simulink model "Radial_LV_Grid_Third"  (R2022a)
settings: Solver=ode23t  StartTime=0.0  StopTime=2  MaxStep=0.1  RelTol=1e-3
libraries: spsThreePhaseVIMeasurementLib x5, spsLoadFlowBusLib x4, spsPower3phPhasorLib x4, spsThreePhaseDynamicLoadLib x3, spsThreePhasePISectionLineLib x2, spsThreePhaseSourceLib x1, spsThreePhaseTransformerTwoWindingsLib x1, spspowerguiLib x1
settings Model: Creator=matm  LastModifiedBy=nikos
settings SolverCC: ShapePreserveControl=EnableAll  AlgebraicLoopSolver=TrustRegion  SolverResetMethod=Robust
settings DataIOCC: ReturnWorkspaceOutputs=off
settings DebuggingCC: SFMachineParentedDataDiag=warning  ArithmeticOperatorsInVariantConditions=warning
settings SFSimCC: SimUseLocalCustomCode=off  CustomCodeUndefinedFunction=UseInterfaceOnly
settings RTWCC: RTWUseLocalCustomCode=off
settings CodeAppCC: StateflowObjectComments=on
settings SimscapeCC: SimscapeNormalizeSystem=off

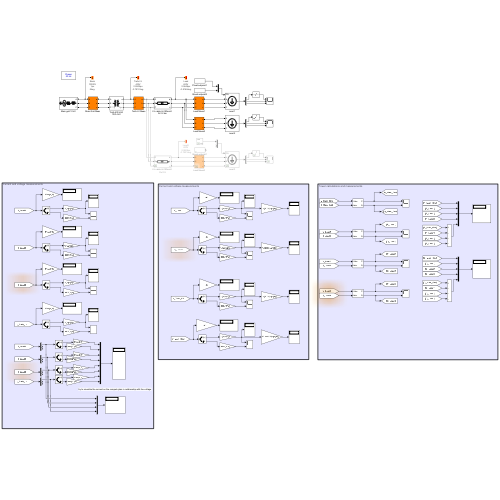
[thumbnail: Simulink's stored preview of the top-level diagram]
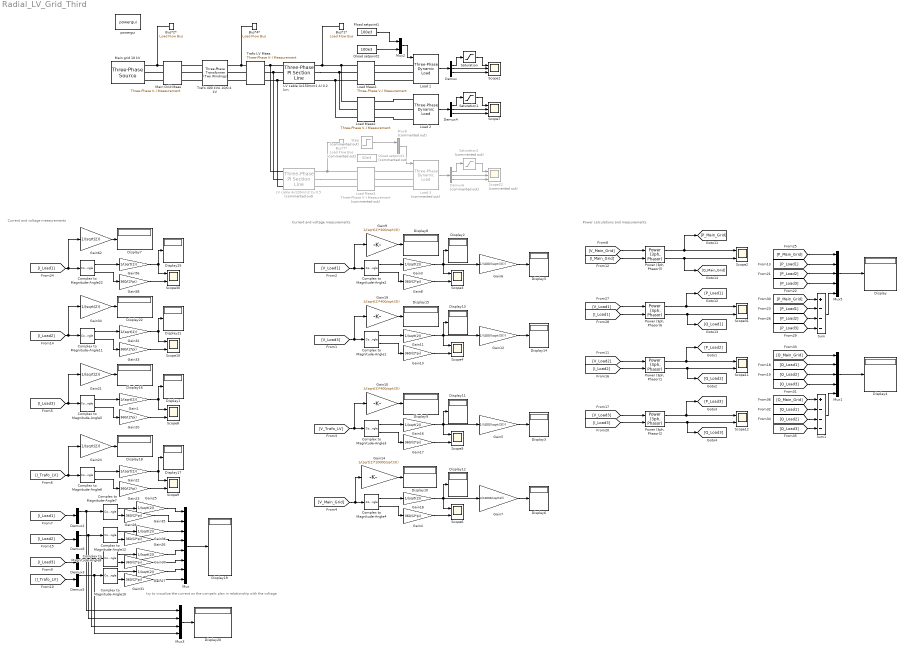
== system Radial_LV_Grid_Third ==
  note: try to visualize the current on the compelx plan in relationship with the voltage
  note: Current and voltage measurements
  note: Power calculations and measurements
  note: Current and voltage measurements
  Bus*1* : spsLoadFlowBusLib/Load Flow Bus  LConnTagsString=a  Phases=single  Connectors=on one side  ID=Load  Vbase=400  Vref=1  Vangle=0  VLF=0.9446  VLFb=1  VLFc=1  angleLF=-0.8162  angleLFb=0  angleLFc=0
      settings: SourceProductBaseCode=PS
  Bus*2* : spsLoadFlowBusLib/Load Flow Bus  LConnTagsString=a  Phases=single  Connectors=on one side  ID=Slack  Vbase=10000  Vref=1  Vangle=0  VLF=1  VLFb=1  VLFc=1  angleLF=0  angleLFb=0  angleLFc=0
      settings: SourceProductBaseCode=PS
  Bus*4* : spsLoadFlowBusLib/Load Flow Bus  LConnTagsString=a  Phases=single  Connectors=on one side  ID=Trafo LV  Vbase=400  Vref=1  Vangle=0  VLF=0.9905  VLFb=1  VLFc=1  angleLF=-0.7817  angleLFb=0  angleLFc=0
      settings: SourceProductBaseCode=PS
  Bus*7* : spsLoadFlowBusLib/Load Flow Bus  Commented=on  LConnTagsString=a  Phases=single  Connectors=on one side  ID=Load3  Vbase=400  Vref=1  Vangle=0  VLF=0.9905  VLFb=1  VLFc=1  angleLF=-0.7821  angleLFb=0  angleLFc=0
      settings: SourceProductBaseCode=PS
  Complex to Magnitude-Angle{1..8,10..12,22} (12 alike) : ComplexToMagnitudeAngle
  Demux{,2..5,8} (6 alike) : Demux  Outputs=3
  Demux6 : Demux  Commented=on  Outputs=3
  Display{,1..22,25} (24 alike) : Display
  Gain{1,3,11,16,18,21..22,24..27,32,34..35,56,62} (16 alike) : Gain  Gain=1/(sqrt(2))
  Gain10 : Gain  Gain=1/(sqrt(2)*400/sqrt(3))
  Gain12 : Gain  Gain=1/(400/(sqrt(3)))
  Gain{4,8,13,17,20,23,28,30..31,33,36,58} (12 alike) : Gain  Gain=360/(2*pi)
  Gain14 : Gain  Gain=1/(sqrt(2)*10000/sqrt(3))
  Gain19 : Gain  Gain=1/(sqrt(2)*400/sqrt(3))
  Gain5 : Gain  Gain=1/(400/(sqrt(3)))
  Gain6 : Gain  Gain=1/(400/(sqrt(3)))
  Gain7 : Gain  Gain=1/(10000/(sqrt(3)))
  Gain9 : Gain  Gain=1/(sqrt(2)*400/sqrt(3))
  LV cable 4x120mm2 Cu 0.5 : spsThreePhasePISectionLineLib/Three-Phase PI Section Line  Commented=on  LConnTagsString=a|b|c  RConnTagsString=A|B|C  Length=0.5  Frequency=50  Resistances=[ 0.1556 0.6224]  Inductances=[ 72e-3/(2*pi*50) 288e-3/(2*pi*50)]  Capacitances=[910e-09 455e-09]
  LV cable 4x150mm2 Al 0.2 km : spsThreePhasePISectionLineLib/Three-Phase PI Section Line  LConnTagsString=a|b|c  RConnTagsString=A|B|C  Length=0.2  Frequency=50  Resistances=[ 0.207 0.828]  Inductances=[ 72e-3/(2*pi*50) 288e-3/(2*pi*50)]  Capacitances=[910e-09 455e-09]
  Load 1 : spsThreePhaseDynamicLoadLib/Three-Phase Dynamic Load  NominalVoltage=[ 0.4e3 50 ]  ActiveReactivePowers=[100000 100e3]  PositiveSequence=[0.944639 -0.816214]  ExternalControl=on  NpNq=[0 0]  TimeConstants="[0  0  0  0]"  MinimumVoltage=0.7  Tfilter=1e-4  LoadFlowParameters=[4 100000 0 0 100000]
      settings: SourceProductBaseCode=PS
  Load 2 : spsThreePhaseDynamicLoadLib/Three-Phase Dynamic Load  NominalVoltage=[ 0.4e3 50 ]  ActiveReactivePowers=[50000 50000]  PositiveSequence=[0.944639 -0.816214]  ExternalControl=off  NpNq=[1 2]  TimeConstants="[0  0  0  0]"  MinimumVoltage=0.7  Tfilter=1e-4  LoadFlowParameters=[4 100000 0 0 100000]
      settings: SourceProductBaseCode=PS
  Load 3 : spsThreePhaseDynamicLoadLib/Three-Phase Dynamic Load  Commented=on  NominalVoltage=[ 0.4e3 50 ]  ActiveReactivePowers=[0 0]  PositiveSequence=[0.990467 -0.782078]  ExternalControl=on  NpNq=[0 0]  TimeConstants="[0  0  0  0]"  MinimumVoltage=0.7  Tfilter=1e-4  LoadFlowParameters=[4 100000 0 0 100000]
      settings: SourceProductBaseCode=PS
  Load Meas1 : spsThreePhaseVIMeasurementLib/Three-Phase V-I Measurement  VoltageMeasurement=phase-to-ground  SetLabelV=on  LabelV=V_Load1  Vpu=off  VpuLL=off  CurrentMeasurement=yes  SetLabelI=on  LabelI=I_Load1  Ipu=off  Pbase=100e6  Vbase=500e3  OutputType=Complex  PhasorSimulation=on  PSBequivalent=0
  Load Meas2 : spsThreePhaseVIMeasurementLib/Three-Phase V-I Measurement  VoltageMeasurement=phase-to-ground  SetLabelV=on  LabelV=V_Load2  Vpu=off  VpuLL=off  CurrentMeasurement=yes  SetLabelI=on  LabelI=I_Load2  Ipu=off  Pbase=100e6  Vbase=500e3  OutputType=Complex  PhasorSimulation=on  PSBequivalent=0
  Load Meas3 : spsThreePhaseVIMeasurementLib/Three-Phase V-I Measurement  Commented=on  VoltageMeasurement=phase-to-ground  SetLabelV=on  LabelV=V_Load3  Vpu=off  VpuLL=off  CurrentMeasurement=yes  SetLabelI=on  LabelI=I_Load3  Ipu=off  Pbase=100e6  Vbase=500e3  OutputType=Complex  PhasorSimulation=on  PSBequivalent=0
  Main Grid Meas : spsThreePhaseVIMeasurementLib/Three-Phase V-I Measurement  VoltageMeasurement=phase-to-ground  SetLabelV=on  LabelV=V_Main_Grid  Vpu=off  VpuLL=off  CurrentMeasurement=yes  SetLabelI=on  LabelI=I_Main_Grid  Ipu=off  Pbase=100e6  Vbase=500e3  OutputType=Complex  PhasorSimulation=on  PSBequivalent=0
  Main grid 10 kV : spsThreePhaseSourceLib/Three-Phase Source  InternalConnection=Yg  VoltagePhases=off  Voltage=(10000)*1.0073  PhaseAngle=0.871  Voltage_phases=[25e3 25e3 25e3]/sqrt(3)  PhaseAngles_phases=[0 -120 +120]  Frequency=50  NonIdealSource=on  SpecifyImpedance=on  Resistance=0.8929  Inductance=16.58e-3  ShortCircuitLevel=10e6  BaseVoltage=10e3  XRratio=10  BusType=swing  Pref=10e3  Qref=0  Prefabc=[10e3, 10e3, 10e3]  Qrefabc=[0, 0, 0]  Qmin=-inf  Qmax=inf
  Mux : Mux  Inputs=8
  Mux1 : Mux  Inputs=5
  Mux2 : Mux  Inputs=2
  Mux3 : Mux
  Mux5 : Mux  Inputs=5
  Mux8 : Mux  Commented=on  Inputs=2
  Pload setpoint1 : Constant  Value=100e3
  Power (3ph, Phasor){1..2,5..6} (4 alike) : spsPower3phPhasorLib/Power (3ph, Phasor)
      settings: SourceProductBaseCode=PS
  Qload setpoint1 : Constant  Commented=on  Value=50e3
  Qload setpoint2 : Constant  Value=100e3
  Saturation : Saturate  UpperLimit=1.15  LowerLimit=0.85
  Saturation1 : Saturate  UpperLimit=1.15  LowerLimit=0.85
  Saturation2 : Saturate  Commented=on  UpperLimit=1.15  LowerLimit=0.85
  Scope1 : Scope  NumInputPorts=3
  Scope{2..6,8..12,30..31} (12 alike) : Scope  NumInputPorts=2
  Scope22 : Scope  Commented=on  NumInputPorts=3
  Scope7 : Scope  NumInputPorts=3
  Step : Step  Commented=on  After=-200e3  SampleTime=0
  Sum : Sum  Inputs=+---
  Sum1 : Sum  Inputs=+---
  Trafo 400 kVA 10/0.4 kV : spsThreePhaseTransformerTwoWindingsLib/Three-Phase Transformer (Two Windings)  Winding1Connection=Yg  Winding2Connection=Yg  CoreType=Three single-phase transformers  SetSaturation=off  Hysteresis=off  DataFile='hysteresis'  SetInitialFlux=off  Measurements=None  UNITS=pu  NominalPower=[ 400e3 , 50 ]  Winding1=[10000 0.0055 0.019]  Winding2=[400 0.0055 0.019]  Rm=500  Lm=500  L0=0.5  Saturation=[0 0;0.0024 1.2;1 1.52]  InitialFluxes=[0.8 -0.8 0.7]  BreakLoop=off  DiscreteSolver=Trapezoidal iterative  DataType=off  TransfoNumber=1
  Trafo LV Meas : spsThreePhaseVIMeasurementLib/Three-Phase V-I Measurement  VoltageMeasurement=phase-to-ground  SetLabelV=on  LabelV=V_Trafo_LV  Vpu=off  VpuLL=off  CurrentMeasurement=yes  SetLabelI=on  LabelI=I_Trafo_LV  Ipu=off  Pbase=100e6  Vbase=500e3  OutputType=Complex  PhasorSimulation=on  PSBequivalent=0
  powergui : spspowerguiLib/powergui  Priority=1  SimulationMode=Phasor  SampleTime=50e-6  frequency=50  Iterations=50  frequencyindice=50  Pbase=1e6  ErrMax=0.0001  UnitsV=kV  UnitsW=kW  buscounter=7  FunctionMessages=off  echomessages=off  EnableUseOfTLC=off  CurrentSourceSwitches=off  DisableSnubberDevices=off  DisableRonSwitches=off  DisableVfSwitches=off  DisplayEquations=off  AutomaticDiscreteSolvers=off  SolverType=Tustin/Backward Euler (TBE)  Interpol=off  ExternalGateDelay=off  methode=off  Ts=10  x0status=blocks  SPID=off  SwTol=0  HookPort=off  NonlinearTolerance=1e-4  nMaxIteration=100  ContinueOnMaxIteration=off  RestoreLinks=warning  ResistiveCurrentMeasurement=off  Frange=[0:2:500]  Ylog=off  Xlog=on  ShowGrid=off  save=off  variable=ZData  structure=ScopeData  ZoomFFT=off  StartTime=0.0  cycles=1  DisplayStyle=1  fundamental=60  FreqAxis=off  MaxFrequency=1000  frequencyindicesteady=1  RmsSteady=2  display=off
  wires:
  Load 1/1 -> Demux/1
  Demux/3 -> Scope1/3
  Demux/2 -> Scope1/2
  Demux/1 -> Saturation/1
  Saturation/1 -> Scope1/1
  Saturation1/1 -> Scope7/1
  Demux4/1 -> Saturation1/1
  Demux4/2 -> Scope7/2
  Demux4/3 -> Scope7/3
  Load 2/1 -> Demux4/1
  Mux2/1 -> Load 1/1
  Mux8/1 -> Load 3/1
  Load 3/1 -> Demux6/1
  Demux6/3 -> Scope22/3
  Demux6/2 -> Scope22/2
  Demux6/1 -> Saturation2/1
  Saturation2/1 -> Scope22/1
  "Power (3ph, Phasor)5"/1 -> Scope2/1, [P_Main_Grid]
  [I_Load1] -> Gain62/1, Complex to Magnitude-Angle22/1
  Complex to Magnitude-Angle22/2 -> Gain58/1
  Gain58/1 -> Scope30/2
  Complex to Magnitude-Angle22/1 -> Gain56/1
  Gain56/1 -> Scope30/1, Display25/1
  [I_Load1] -> "Power (3ph, Phasor)6"/2
  "Power (3ph, Phasor)5"/2 -> Scope2/2, [Q_Main_Grid]
  Mux5/1 -> Display/1
  [V_Main_Grid] -> "Power (3ph, Phasor)5"/1
  [I_Main_Grid] -> "Power (3ph, Phasor)5"/2
  "Power (3ph, Phasor)6"/2 -> [Q_Load1], Scope31/2
  [V_Load1] -> "Power (3ph, Phasor)6"/1
  "Power (3ph, Phasor)6"/1 -> [P_Load1], Scope31/1
  Gain62/1 -> Display7/1
  Gain6/1 -> Display5/1
  Gain8/1 -> Scope3/2
  Complex to Magnitude-Angle2/1 -> Gain3/1
  Gain7/1 -> Display6/1
  Gain5/1 -> Display3/1
  Complex to Magnitude-Angle3/2 -> Gain17/1
  Gain17/1 -> Scope5/2
  Gain3/1 -> Scope3/1, Gain6/1, Display2/1
  Complex to Magnitude-Angle2/2 -> Gain8/1
  [V_Load1] -> Gain9/1, Complex to Magnitude-Angle2/1
  Gain18/1 -> Scope6/1, Gain7/1, Display12/1
  Complex to Magnitude-Angle3/1 -> Gain16/1
  [V_Main_Grid] -> Gain14/1, Complex to Magnitude-Angle4/1
  Gain16/1 -> Gain5/1, Scope5/1, Display11/1
  Complex to Magnitude-Angle4/2 -> Gain4/1
  Gain4/1 -> Scope6/2
  Gain14/1 -> Display10/1
  Complex to Magnitude-Angle4/1 -> Gain18/1
  Gain9/1 -> Display8/1
  Gain10/1 -> Display9/1
  [V_Trafo_LV] -> Gain10/1, Complex to Magnitude-Angle3/1
  [V_Load3] -> Gain19/1, Complex to Magnitude-Angle1/1
  Gain11/1 -> Scope4/1, Gain12/1, Display13/1
  Complex to Magnitude-Angle1/2 -> Gain13/1
  Gain12/1 -> Display14/1
  Gain13/1 -> Scope4/2
  Complex to Magnitude-Angle1/1 -> Gain11/1
  Gain19/1 -> Display15/1
  Gain21/1 -> Display16/1
  Gain1/1 -> Display1/1, Scope8/1
  Complex to Magnitude-Angle5/1 -> Gain1/1
  Gain20/1 -> Scope8/2
  Complex to Magnitude-Angle5/2 -> Gain20/1
  [I_Load3] -> Complex to Magnitude-Angle5/1, Gain21/1
  [I_Trafo_LV] -> Gain24/1, Complex to Magnitude-Angle6/1
  Complex to Magnitude-Angle6/2 -> Gain23/1
  Gain23/1 -> Scope9/2
  Complex to Magnitude-Angle6/1 -> Gain22/1
  Gain22/1 -> Scope9/1, Display17/1
  Gain24/1 -> Display18/1
  [I_Load1] -> Demux2/1
  [I_Load3] -> Demux3/1
  [I_Trafo_LV] -> Demux5/1
  Demux2/1 -> Mux3/1, Complex to Magnitude-Angle7/1
  Complex to Magnitude-Angle7/1 -> Gain25/1
  Complex to Magnitude-Angle7/2 -> Gain28/1
  Demux3/1 -> Mux3/3, Complex to Magnitude-Angle8/1
  Complex to Magnitude-Angle8/1 -> Gain26/1
  Complex to Magnitude-Angle8/2 -> Gain30/1
  Demux5/1 -> Mux3/4, Complex to Magnitude-Angle10/1
  Complex to Magnitude-Angle10/1 -> Gain27/1
  Complex to Magnitude-Angle10/2 -> Gain31/1
  Mux/1 -> Display19/1
  Mux3/1 -> Display20/1
  [I_Load2] -> Gain34/1, Complex to Magnitude-Angle11/1
  Complex to Magnitude-Angle11/2 -> Gain33/1
  Gain33/1 -> Scope10/2
  Complex to Magnitude-Angle11/1 -> Gain32/1
  Gain32/1 -> Scope10/1, Display21/1
  Gain34/1 -> Display22/1
  Complex to Magnitude-Angle12/2 -> Gain36/1
  Complex to Magnitude-Angle12/1 -> Gain35/1
  Demux8/1 -> Mux3/2, Complex to Magnitude-Angle12/1
  [I_Load2] -> Demux8/1
  Gain25/1 -> Mux/1
  Gain28/1 -> Mux/2
  Gain35/1 -> Mux/3
  Gain36/1 -> Mux/4
  Gain26/1 -> Mux/5
  Gain30/1 -> Mux/6
  Gain27/1 -> Mux/7
  Gain31/1 -> Mux/8
  "Power (3ph, Phasor)1"/1 -> Scope11/1, [P_Load2]
  [V_Load2] -> "Power (3ph, Phasor)1"/1
  "Power (3ph, Phasor)1"/2 -> Scope11/2, [Q_Load2]
  [I_Load2] -> "Power (3ph, Phasor)1"/2
  [I_Load3] -> "Power (3ph, Phasor)2"/2
  "Power (3ph, Phasor)2"/2 -> [Q_Load3], Scope12/2
  [V_Load3] -> "Power (3ph, Phasor)2"/1
  "Power (3ph, Phasor)2"/1 -> [P_Load3], Scope12/1
  [P_Main_Grid] -> Mux5/1
  [P_Load1] -> Mux5/2
  [P_Load2] -> Mux5/3
  [P_Load3] -> Mux5/4
  [P_Main_Grid] -> Sum/1
  [P_Load2] -> Sum/3
  [P_Load1] -> Sum/2
  [P_Load3] -> Sum/4
  Sum/1 -> Mux5/5
  Sum1/1 -> Mux1/5
  [Q_Load3] -> Sum1/4
  [Q_Load1] -> Sum1/2
  [Q_Load2] -> Sum1/3
  [Q_Main_Grid] -> Sum1/1
  [Q_Load3] -> Mux1/4
  [Q_Load2] -> Mux1/3
  [Q_Load1] -> Mux1/2
  [Q_Main_Grid] -> Mux1/1
  Mux1/1 -> Display4/1
  Pload setpoint1/1 -> Mux2/1
  Step/1 -> Mux8/1
  Qload setpoint2/1 -> Mux2/2
  connections:
  Main grid 10 kV/RConn1 -- Main Grid Meas/LConn1 -- Bus*2*/LConn1
  Main Grid Meas/LConn2 -- Main grid 10 kV/RConn2
  Main Grid Meas/LConn3 -- Main grid 10 kV/RConn3
  Trafo 400 kVA 10/0.4 kV/LConn3 -- Main Grid Meas/RConn3
  Trafo 400 kVA 10/0.4 kV/LConn1 -- Main Grid Meas/RConn1
  Trafo 400 kVA 10/0.4 kV/LConn2 -- Main Grid Meas/RConn2
  Trafo 400 kVA 10/0.4 kV/RConn1 -- Trafo LV Meas/LConn1 -- Bus*4*/LConn1
  Trafo LV Meas/LConn2 -- Trafo 400 kVA 10/0.4 kV/RConn2
  Trafo LV Meas/LConn3 -- Trafo 400 kVA 10/0.4 kV/RConn3
  LV cable 4x150mm2 Al 0.2 km/LConn1 -- LV cable 4x120mm2 Cu 0.5/LConn1 -- Trafo LV Meas/RConn1
  LV cable 4x150mm2 Al 0.2 km/LConn3 -- LV cable 4x120mm2 Cu 0.5/LConn3 -- Trafo LV Meas/RConn3
  LV cable 4x150mm2 Al 0.2 km/RConn1 -- Bus*1*/LConn1 -- Load Meas2/LConn1 -- Load Meas1/LConn1
  LV cable 4x150mm2 Al 0.2 km/RConn2 -- Load Meas2/LConn2 -- Load Meas1/LConn2
  Load Meas1/LConn3 -- Load Meas2/LConn3 -- LV cable 4x150mm2 Al 0.2 km/RConn3
  Load 1/LConn3 -- Load Meas1/RConn3
  Load 1/LConn2 -- Load Meas1/RConn2
  Load 1/LConn1 -- Load Meas1/RConn1
  Load 2/LConn1 -- Load Meas2/RConn1
  Load 2/LConn2 -- Load Meas2/RConn2
  Load 2/LConn3 -- Load Meas2/RConn3
  Load Meas3/LConn1 -- Bus*7*/LConn1 -- LV cable 4x120mm2 Cu 0.5/RConn1
  Load Meas3/LConn3 -- LV cable 4x120mm2 Cu 0.5/RConn3
  LV cable 4x120mm2 Cu 0.5/RConn2 -- Load Meas3/LConn2
  Load 3/LConn1 -- Load Meas3/RConn1
  Load 3/LConn2 -- Load Meas3/RConn2
  Load 3/LConn3 -- Load Meas3/RConn3
  Trafo LV Meas/RConn2 -- LV cable 4x120mm2 Cu 0.5/LConn2 -- LV cable 4x150mm2 Al 0.2 km/LConn2
